simulink model "ex_13_model"  (R2014a)
settings: Solver=ode45  StartTime=0.0  StopTime=10.0  RelTol=1e-3
values from neighbouring files (symbols this model uses):
  G = 0    [ex_13_init.m]
  x = -(1/J) * (a + (K^2/R))    (= -20.4)    [ex_13_init.m]
  y = (K/(J*R))    (= 400)    [ex_13_init.m]
  z = -(1/J)    (= -4000)    [ex_13_init.m]
undefined symbols (not defined in the file or in its folder): Kp
settings Model: Creator=Nino  LastModifiedBy=Nino

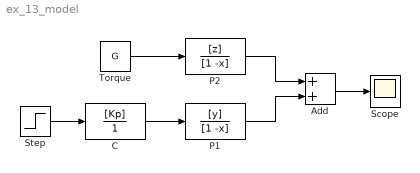
== system ex_13_model ==
  Add : Sum
  C : TransferFcn  Numerator=[Kp]  Denominator=[1]
  P1 : TransferFcn  Numerator=[y]  Denominator=[1 -x]
  P2 : TransferFcn  Numerator=[z]  Denominator=[1 -x]
  Scope : Scope
  Step : Step  After=10  SampleTime=0
  Torque : Constant  Value=G
  wires:
  Add/1 -> Scope/1
  Torque/1 -> P2/1
  P2/1 -> Add/1
  P1/1 -> Add/2
  C/1 -> P1/1
  Step/1 -> C/1
